simulink model "SimulinkSimples"  (R2013b)
settings: Solver=ode3  StartTime=0.0  StopTime=20  RelTol=1e-3
values from neighbouring files (symbols this model uses):
  Ad = G_disc.a    [InicializaSimples.m]
  Bd = G_disc.b    [InicializaSimples.m]
  C = [1 0]    [InicializaSimples.m]
settings Model: Creator=ThiagoCordeiro  LastModifiedBy=ThiagoFelippe

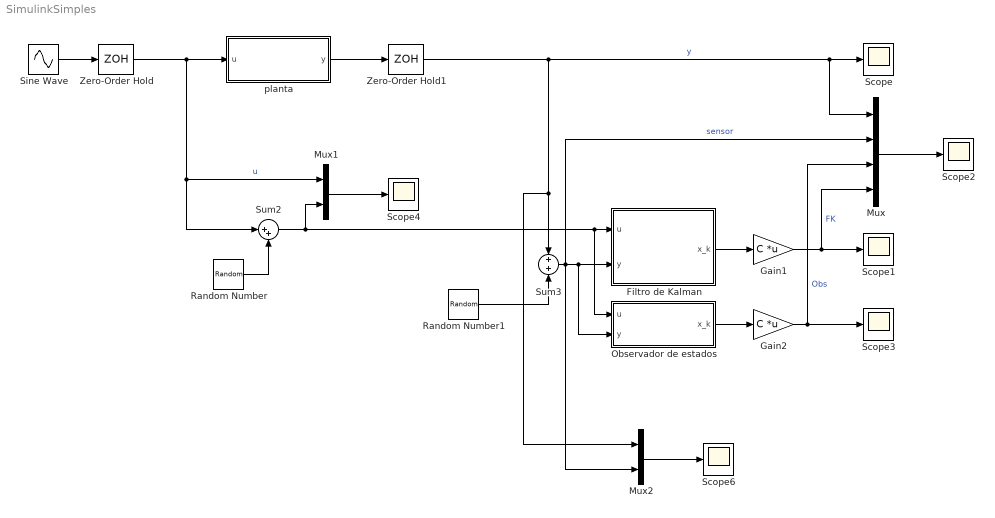
== system SimulinkSimples ==
  Filtro de Kalman : Subsystem
  Gain1 : Gain  Gain=C  Multiplication=Matrix(K*u)
  Gain2 : Gain  Gain=C  Multiplication=Matrix(K*u)
  Mux : Mux
  Mux1 : Mux  Inputs=2
  Mux2 : Mux  Inputs=2
  Observador de estados : Subsystem
  Random Number : RandomNumber  Seed=round(rand(1)*(2^32-1))  SampleTime=0.01
  Random Number1 : RandomNumber  Seed=round(rand(1)*(2^32-1))  SampleTime=0.01
  Scope{,1..4,6} (6 alike) : Scope
      Scope2 settings: ShowLegends=on  SaveName=ScopeData2
      Scope3 settings: SaveName=ScopeData4
      Scope4 settings: SaveName=ScopeData6
      Scope6 settings: SaveName=ScopeData8
  Sine Wave : Sin  Phase=pi/2  SampleTime=0
  Sum2 : Sum  Inputs=|++
  Sum3 : Sum  Inputs=+|+
  Zero-Order Hold : ZeroOrderHold  SampleTime=0.01
  Zero-Order Hold1 : ZeroOrderHold  SampleTime=0.01
  planta : Subsystem
  wires:
  Filtro de Kalman/1(x_k) -> Gain1/1
  Gain1/1 -> Mux/4, Scope1/1  "FK"
  Mux/1 -> Scope2/1
  Zero-Order Hold/1 -> planta/1(u), Mux1/1, Sum2/1  "u"
  Sum2/1 -> Mux1/2, Observador de estados/1(u), Filtro de Kalman/1(u)
  Random Number/1 -> Sum2/2
  Sum3/1 -> Mux2/2, Mux/2, Observador de estados/2(y), Filtro de Kalman/2(y)  "sensor"
  Random Number1/1 -> Sum3/2
  Observador de estados/1(x_k) -> Gain2/1
  Gain2/1 -> Scope3/1, Mux/3  "Obs"
  planta/1(y) -> Zero-Order Hold1/1
  Sine Wave/1 -> Zero-Order Hold/1
  Mux1/1 -> Scope4/1
  Mux2/1 -> Scope6/1
  Zero-Order Hold1/1 -> Mux/1, Scope/1, Mux2/1, Sum3/1  "y"

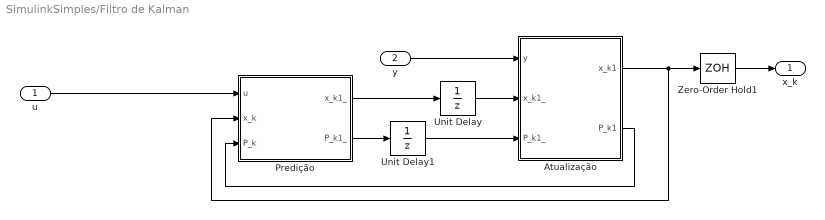
== system SimulinkSimples/Filtro de Kalman ==
  u : Inport
  y : Inport  Port=2
  Atualização : Subsystem
  Predição : Subsystem
  Unit Delay : UnitDelay  InitialCondition=[0.7;-0.7]*0 + randn(2,1)  SampleTime=0.01
  Unit Delay1 : UnitDelay  InitialCondition=1*eye(2)  SampleTime=0.01
  Zero-Order Hold1 : ZeroOrderHold  SampleTime=0.01
  x_k : Outport
  wires:
  u/1 -> Predição/1(u)
  y/1 -> Atualização/1(y)
  Atualização/1(x_k1) -> Predição/2(x_k), Zero-Order Hold1/1
  Atualização/2(P_k1) -> Predição/3(P_k)
  Zero-Order Hold1/1 -> x_k/1
  Predição/2(P_k1_) -> Unit Delay1/1
  Unit Delay1/1 -> Atualização/3(P_k1_)
  Unit Delay/1 -> Atualização/2(x_k1_)
  Predição/1(x_k1_) -> Unit Delay/1

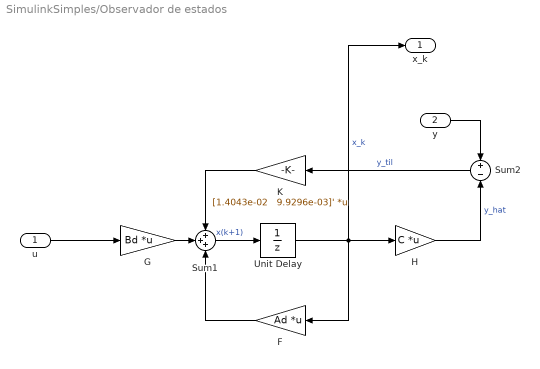
== system SimulinkSimples/Observador de estados ==
  u : Inport
  y : Inport  Port=2
  F : Gain  Gain=Ad  Multiplication=Matrix(K*u)
  G : Gain  Gain=Bd  Multiplication=Matrix(K*u)
  H : Gain  Gain=C  Multiplication=Matrix(K*u)
  K : Gain  Gain="[1.4043e-02   9.9296e-03]'"  Multiplication=Matrix(K*u)
  Sum1 : Sum  Inputs=+++
  Sum2 : Sum  Inputs=+|-
  Unit Delay : UnitDelay  InitialCondition=[0.7;-0.7]*0  SampleTime=-1
  x_k : Outport
  wires:
  Sum1/1 -> Unit Delay/1  "x(k+1)"
  Unit Delay/1 -> F/1, H/1, x_k/1  "x_k"
  u/1 -> G/1
  G/1 -> Sum1/2
  F/1 -> Sum1/3
  y/1 -> Sum2/1
  H/1 -> Sum2/2  "y_hat"
  Sum2/1 -> K/1  "y_til"
  K/1 -> Sum1/1

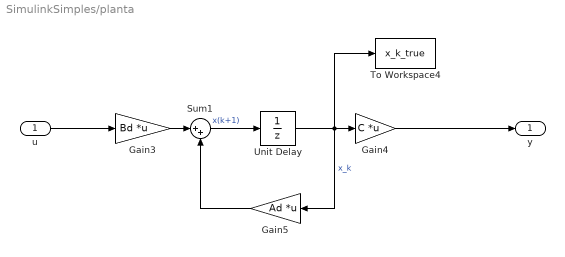
== system SimulinkSimples/planta ==
  u : Inport
  Gain3 : Gain  Gain=Bd  Multiplication=Matrix(K*u)
  Gain4 : Gain  Gain=C  Multiplication=Matrix(K*u)
  Gain5 : Gain  Gain=Ad  Multiplication=Matrix(K*u)
  Sum1 : Sum  Inputs=|++
  To Workspace4 : ToWorkspace  VariableName=x_k_true  SampleTime=-1  SaveFormat=Timeseries
  Unit Delay : UnitDelay  InitialCondition=[0;0]  SampleTime=-1
  y : Outport
  wires:
  Gain3/1 -> Sum1/1
  Sum1/1 -> Unit Delay/1  "x(k+1)"
  Unit Delay/1 -> To Workspace4/1, Gain4/1, Gain5/1  "x_k"
  Gain5/1 -> Sum1/2
  u/1 -> Gain3/1
  Gain4/1 -> y/1

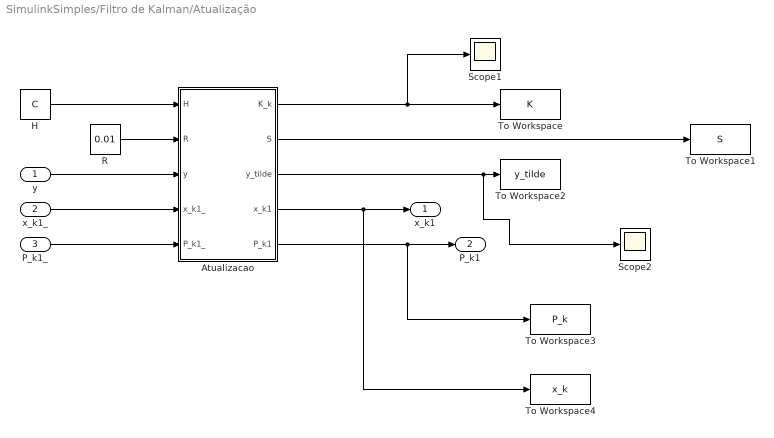
== system SimulinkSimples/Filtro de Kalman/Atualização ==
  y : Inport
  x_k1_ : Inport  Port=2
  P_k1_ : Inport  Port=3
  Atualizacao : MATLAB Function  TreatAsAtomicUnit=on  SystemSampleTime=0.01
  H : Constant  Value=C  VectorParams1D=off
  R : Constant  Value=0.01
  Scope1 : Scope
      settings: SaveName=ScopeData3
  Scope2 : Scope
      settings: SaveName=ScopeData5
  To Workspace : ToWorkspace  VariableName=K  SampleTime=-1  SaveFormat=Timeseries
  To Workspace1 : ToWorkspace  VariableName=S  SampleTime=-1  SaveFormat=Timeseries
  To Workspace2 : ToWorkspace  VariableName=y_tilde  SampleTime=-1  SaveFormat=Timeseries
  To Workspace3 : ToWorkspace  VariableName=P_k  SampleTime=-1  SaveFormat=Timeseries
  To Workspace4 : ToWorkspace  VariableName=x_k  SampleTime=-1  SaveFormat=Timeseries
  x_k1 : Outport
  P_k1 : Outport  Port=2
  wires:
  y/1 -> Atualizacao/3(y)
  x_k1_/1 -> Atualizacao/4(x_k1_)
  P_k1_/1 -> Atualizacao/5(P_k1_)
  Atualizacao/4(x_k1) -> To Workspace4/1, x_k1/1
  Atualizacao/5(P_k1) -> To Workspace3/1, P_k1/1
  H/1 -> Atualizacao/1(H)
  R/1 -> Atualizacao/2(R)
  Atualizacao/1(K_k) -> Scope1/1, To Workspace/1
  Atualizacao/2(S) -> To Workspace1/1
  Atualizacao/3(y_tilde) -> Scope2/1, To Workspace2/1

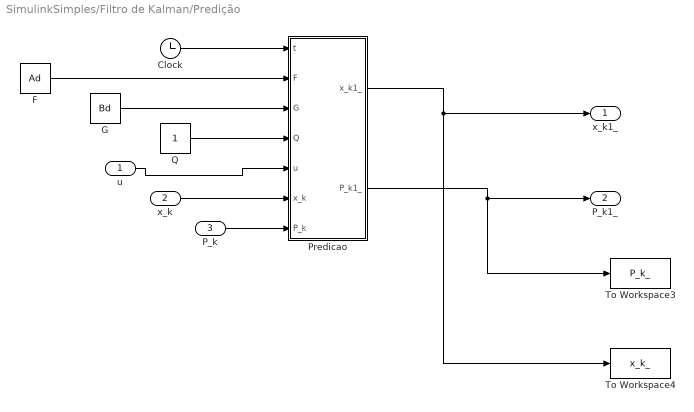
== system SimulinkSimples/Filtro de Kalman/Predição ==
  u : Inport
  x_k : Inport  Port=2
  P_k : Inport  Port=3
  Clock : Clock
  F : Constant  Value=Ad
  G : Constant  Value=Bd  VectorParams1D=off
  Predicao : MATLAB Function  TreatAsAtomicUnit=on  SystemSampleTime=0.01
  Q : Constant
  To Workspace3 : ToWorkspace  VariableName=P_k_  SampleTime=-1  SaveFormat=Timeseries
  To Workspace4 : ToWorkspace  VariableName=x_k_  SampleTime=-1  SaveFormat=Timeseries
  x_k1_ : Outport
  P_k1_ : Outport  Port=2
  wires:
  u/1 -> Predicao/5(u)
  x_k/1 -> Predicao/6(x_k)
  P_k/1 -> Predicao/7(P_k)
  F/1 -> Predicao/2(F)
  G/1 -> Predicao/3(G)
  Q/1 -> Predicao/4(Q)
  Predicao/1(x_k1_) -> To Workspace4/1, x_k1_/1
  Predicao/2(P_k1_) -> To Workspace3/1, P_k1_/1
  Clock/1 -> Predicao/1(t)

== matlab function SimulinkSimples/Filtro de Kalman/Atualização/Atualizacao ==
  data: H input; R input; K_k output; S output; y_tilde output; y input; x_k1_ input; P_k1_ input; x_k1 output; P_k1 output
function [K_k, S, y_tilde, x_k1, P_k1] = fcn(H, R, y, x_k1_, P_k1_)
%#codegen

% Trecho abaixo nao depende nem do estado estimado, nem da medida obtida,
% entao pode ser calculado offline e armazenado em tabela
S = H * P_k1_ * H' + R;
Pxy = P_k1_ * H';
K_k  =  Pxy / S;
KH = K_k*H;
I = eye(size(KH));
I_KH = I - KH;
P_k1 = I_KH * P_k1_ * I_KH' + K_k * R * K_k';
% --- fim do trecho que pode ser calculado offline

y_hat = H * x_k1_;
y_tilde = y - y_hat;
x_k1 = x_k1_ + K_k * y_tilde;

== matlab function SimulinkSimples/Filtro de Kalman/Predição/Predicao ==
  data: t input; F input; G input; Q input; u input; x_k1_ output; x_k input; P_k input; P_k1_ output
function [x_k1_,P_k1_] = fcn(t, F, G, Q, u, x_k, P_k)
%#codegen
if t >= 0
    x_k1_ = F*x_k + G*u;
    P_k1_ = F*P_k*F' + G*Q*G';
else %inicializacao
    x_k1_ = x_k;
    P_k1_ = P_k;
end
